simulink model "Glide_flare_alt"  (R2020a)
settings: Solver=VariableStepAuto  StartTime=0.0  StopTime=300  RelTol=1e-3
values from neighbouring files (symbols this model uses):
  A_reduced = A_lo([3,7,8,5,11],[3,7,8,5,11])    [landing.m]
  B_reduced = A_lo([3,7,8,5,11], [13,14])    [landing.m]
  C_reduced = C_lo([3,7,8,5,11],[3,7,8,5,11])    [landing.m]
  D_reduced = D_lo([3,7,8,5,11], [1,2])    [landing.m]
  elevator = -0.09    [FindF16Dynamics.m]    (also in runF16Sim.m; runLINF16sim.m)
  thrust = 5000    [FindF16Dynamics.m]    (also in landing.m = 2826.8165; runF16Sim.m; runLINF16sim.m = 0)
undefined symbols (not defined in the file or in its folder): magnitude
libraries: simulink_extras x5
settings Model: SnapshotBufferSize=10000  Creator=sarka  LastModifiedBy=mbrum

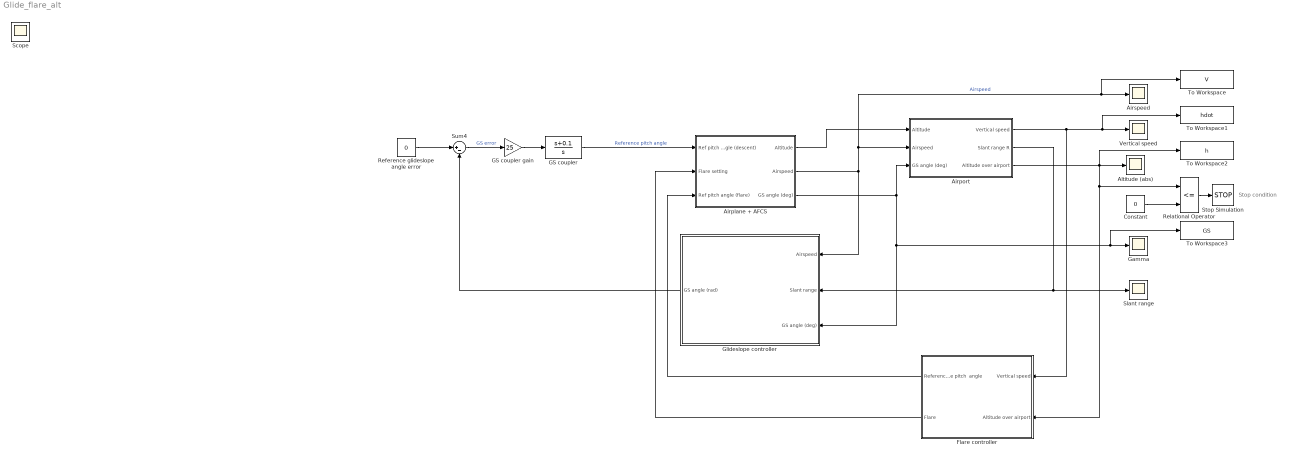
== system Glide_flare_alt ==
  note: Stop condition
  Airplane + AFCS : Subsystem
  Airport : Subsystem
  Airspeed : Scope
  Altitude (abs) : Scope
  Constant : Constant  Value=0
  Flare controller : Subsystem
  GS coupler : TransferFcn  Numerator=[1 0.1]  Denominator=[1 0]
  GS coupler gain : Gain  Gain=25
  Gamma : Scope
  Glideslope controller : Subsystem
  Reference glideslope angle error : Constant  Value=0
  Relational Operator : RelationalOperator  Operator=<=  OutDataTypeStr=boolean  RndMeth=Simplest
  Slant range : Scope
  Stop Simulation : Stop
  Sum4 : Sum  Inputs=|+-
  To Workspace : ToWorkspace  VariableName=V  SampleTime=-1
  To Workspace1 : ToWorkspace  VariableName=hdot  SampleTime=-1
  To Workspace2 : ToWorkspace  VariableName=h  SampleTime=-1
  To Workspace3 : ToWorkspace  VariableName=GS  SaveFormat=Timeseries  SampleTime=-1
  Vertical speed : Scope
  Scope : Scope
  wires:
  Airplane + AFCS/2(Airspeed) -> To Workspace/1, Airspeed/1, Airport/2(Airspeed), Glideslope controller/1(Airspeed)  "Airspeed"
  Airplane + AFCS/3(GS angle (deg)) -> Airport/3(GS angle (deg)), Glideslope controller/3(GS angle (deg)), To Workspace3/1, Gamma/1
  Airport/1(Vertical speed) -> To Workspace1/1, Vertical speed/1, Flare controller/1(Vertical speed)
  Reference glideslope angle error/1 -> Sum4/1
  Glideslope controller/1(GS angle (rad)) -> Sum4/2
  Sum4/1 -> GS coupler gain/1  "GS error"
  GS coupler gain/1 -> GS coupler/1
  Airplane + AFCS/1(Altitude) -> Airport/1(Altitude)
  Airport/2(Slant range R) -> Glideslope controller/2(Slant range), Slant range/1
  GS coupler/1 -> Airplane + AFCS/1(Ref pitch angle (descent))  "Reference pitch angle"
  Flare controller/2(Flare) -> Airplane + AFCS/2(Flare setting)
  Flare controller/1(Reference pitch  angle) -> Airplane + AFCS/3(Ref pitch angle (flare))
  Airport/3(Altitude over airport) -> To Workspace2/1, Flare controller/2(Altitude over airport), Relational Operator/1, Altitude (abs)/1
  Constant/1 -> Relational Operator/2
  Relational Operator/1 -> Stop Simulation/1

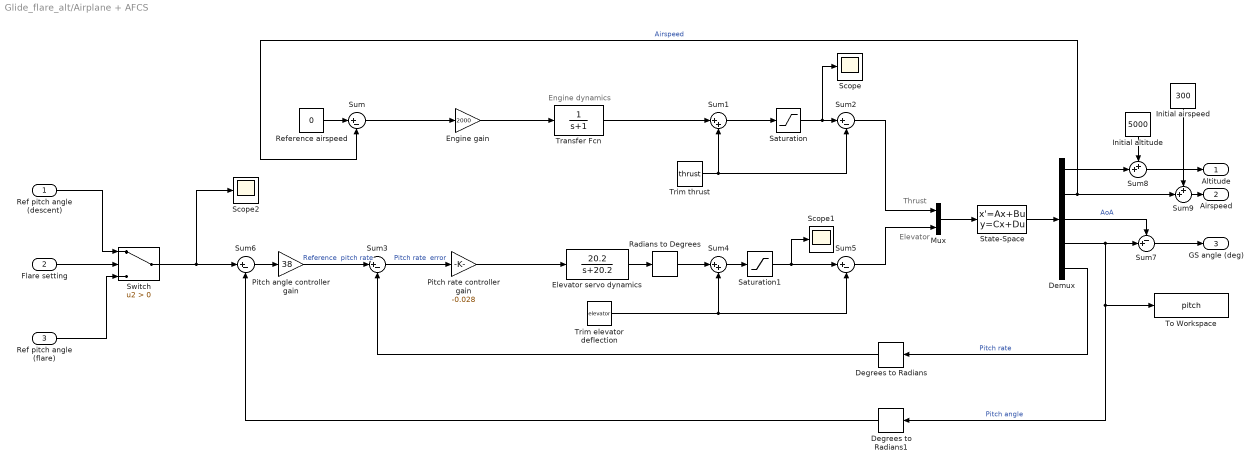
== system Glide_flare_alt/Airplane + AFCS ==
  note: Engine dynamics
  note: Elevator
  note: Thrust
  Ref pitch angle (descent) : Inport
  Flare setting : Inport  Port=2
  Ref pitch angle (flare) : Inport  Port=3
  Degrees to Radians : simulink_extras/Transformations/Degrees to Radians
  Degrees to Radians1 : simulink_extras/Transformations/Degrees to Radians
  Demux : Demux  Outputs=5
  Elevator servo dynamics : TransferFcn  Numerator=[20.2]  Denominator=[1 20.2]
  Engine gain : Gain  Gain=2000
  Initial airspeed : Constant  Value=300
  Initial altitude : Constant  Value=5000
  Mux : Mux  Inputs=2
  Pitch angle controller gain : Gain  Gain=38
  Pitch rate controller gain : Gain  Gain=-0.028
  Radians to Degrees : simulink_extras/Transformations/Radians to Degrees
  Reference airspeed : Constant  Value=0
  Saturation : Saturate  UpperLimit=19000  LowerLimit=1000
  Saturation1 : Saturate  UpperLimit=25  LowerLimit=-25
  Scope : Scope
  Scope1 : Scope
  Scope2 : Scope
  State-Space : StateSpace  A=A_reduced  B=B_reduced  C=C_reduced  D=D_reduced  InitialCondition=0
  Sum{,2..3,5..6} (5 alike) : Sum  Inputs=|+-
  Sum1 : Sum  Inputs=|++
  Sum4 : Sum  Inputs=|++
  Sum7 : Sum  Inputs=-+|
  Sum8 : Sum  Inputs=++|
  Sum9 : Sum  Inputs=++|
  Switch : Switch  Criteria=u2 > Threshold
  To Workspace : ToWorkspace  VariableName=pitch  SaveFormat=Timeseries  SampleTime=-1
  Transfer Fcn : TransferFcn  Denominator=[1 1]
  Trim elevator deflection : Constant  Value=elevator
  Trim thrust : Constant  Value=thrust
  Altitude : Outport
  Airspeed : Outport  Port=2
  GS angle (deg) : Outport  Port=3
  wires:
  Sum/1 -> Engine gain/1
  Radians to Degrees/1 -> Sum4/1
  Mux/1 -> State-Space/1
  Sum1/1 -> Saturation/1
  Pitch rate controller gain/1 -> Elevator servo dynamics/1
  Transfer Fcn/1 -> Sum1/1
  Sum4/1 -> Saturation1/1
  Elevator servo dynamics/1 -> Radians to Degrees/1
  Saturation/1 -> Scope/1, Sum2/1
  Sum2/1 -> Mux/1
  Trim elevator deflection/1 -> Sum4/2, Sum5/2
  Sum5/1 -> Mux/2
  Trim thrust/1 -> Sum2/2, Sum1/2
  Saturation1/1 -> Sum5/1, Scope1/1
  Reference airspeed/1 -> Sum/1
  Sum3/1 -> Pitch rate controller gain/1  "Pitch rate  error"
  Pitch angle controller gain/1 -> Sum3/1  "Reference  pitch rate"
  Engine gain/1 -> Transfer Fcn/1
  Demux/5 -> Degrees to Radians/1  "Pitch rate"
  Sum6/1 -> Pitch angle controller gain/1
  Demux/4 -> Degrees to Radians1/1, To Workspace/1, Sum7/2  "Pitch angle"
  State-Space/1 -> Demux/1
  Demux/3 -> Sum7/1  "AoA"
  Demux/1 -> Sum8/2
  Sum7/1 -> GS angle (deg)/1
  Degrees to Radians1/1 -> Sum6/2
  Degrees to Radians/1 -> Sum3/2
  Sum8/1 -> Altitude/1
  Initial altitude/1 -> Sum8/1
  Sum9/1 -> Airspeed/1
  Demux/2 -> Sum/2, Sum9/2  "Airspeed"
  Initial airspeed/1 -> Sum9/1
  Ref pitch angle (descent)/1 -> Switch/1
  Flare setting/1 -> Switch/2
  Ref pitch angle (flare)/1 -> Switch/3
  Switch/1 -> Scope2/1, Sum6/1

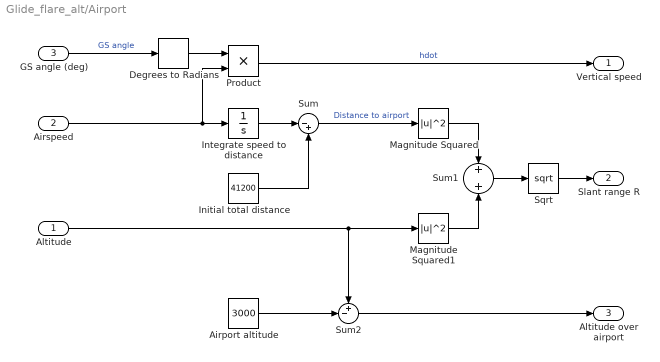
== system Glide_flare_alt/Airport ==
  Altitude : Inport
  Airspeed : Inport  Port=2
  GS angle (deg) : Inport  Port=3
  Airport altitude : Constant  Value=3000
  Degrees to Radians : simulink_extras/Transformations/Degrees to Radians
  Initial total distance : Constant  Value=41200
  Integrate speed to distance : Integrator
  Magnitude Squared : Math  Operator=magnitude^2  SaturateOnIntegerOverflow=on
  Magnitude Squared1 : Math  Operator=magnitude^2  SaturateOnIntegerOverflow=on
  Product : Product
  Sqrt : Sqrt  SaturateOnIntegerOverflow=on
  Sum : Sum  Inputs=|-+
  Sum1 : Sum  Inputs=+|+
  Sum2 : Sum  Inputs=+-|
  Vertical speed : Outport
  Slant range R : Outport  Port=2
  Altitude over airport : Outport  Port=3
  wires:
  GS angle (deg)/1 -> Degrees to Radians/1  "GS angle"
  Airspeed/1 -> Integrate speed to distance/1, Product/2
  Degrees to Radians/1 -> Product/1
  Product/1 -> Vertical speed/1  "hdot"
  Initial total distance/1 -> Sum/2
  Integrate speed to distance/1 -> Sum/1
  Sum/1 -> Magnitude Squared/1  "Distance to airport"
  Altitude/1 -> Sum2/1, Magnitude Squared1/1
  Sum1/1 -> Sqrt/1
  Magnitude Squared/1 -> Sum1/1
  Magnitude Squared1/1 -> Sum1/2
  Sqrt/1 -> Slant range R/1
  Airport altitude/1 -> Sum2/2
  Sum2/1 -> Altitude over airport/1

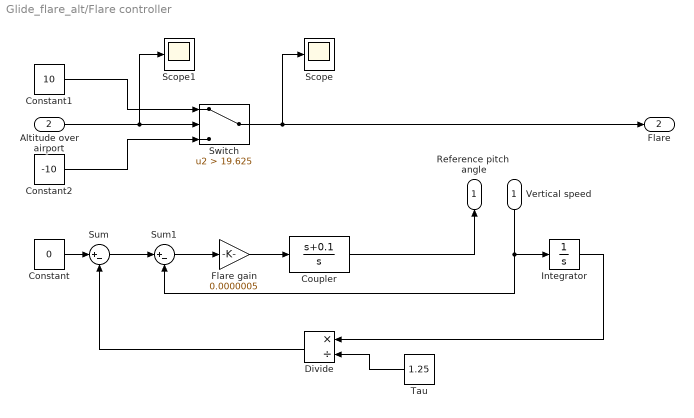
== system Glide_flare_alt/Flare controller ==
  Vertical speed : Inport
  Altitude over airport : Inport  Port=2
  Constant : Constant  Value=0
  Constant1 : Constant  Value=10
  Constant2 : Constant  Value=-10
  Coupler : TransferFcn  Numerator=[1 0.1]  Denominator=[1 0]
  Divide : Product  Inputs=*/
  Flare gain : Gain  Gain=0.0000005
  Integrator : Integrator
  Scope : Scope
  Scope1 : Scope
  Sum : Sum  Inputs=|+-
  Sum1 : Sum  Inputs=|+-
  Switch : Switch  Criteria=u2 > Threshold  Threshold=19.625
  Tau : Constant  Value=1.25
  Reference pitch  angle : Outport
  Flare : Outport  Port=2
  wires:
  Vertical speed/1 -> Sum1/2, Integrator/1
  Integrator/1 -> Divide/1
  Constant/1 -> Sum/1
  Sum/1 -> Sum1/1
  Flare gain/1 -> Coupler/1
  Sum1/1 -> Flare gain/1
  Coupler/1 -> Reference pitch  angle/1
  Altitude over airport/1 -> Scope1/1, Switch/2
  Constant1/1 -> Switch/1
  Constant2/1 -> Switch/3
  Switch/1 -> Scope/1, Flare/1
  Divide/1 -> Sum/2
  Tau/1 -> Divide/2

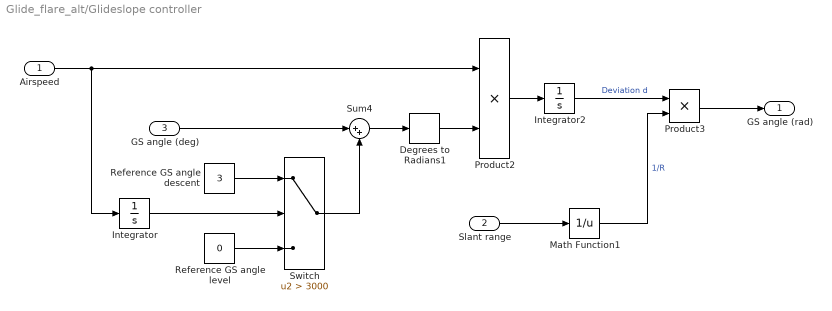
== system Glide_flare_alt/Glideslope controller ==
  Airspeed : Inport
  Slant range : Inport  Port=2
  GS angle (deg) : Inport  Port=3
  Degrees to Radians1 : simulink_extras/Transformations/Degrees to Radians
  Integrator : Integrator
  Integrator2 : Integrator
  Math Function1 : Math  Operator=reciprocal  SignedPower=on  RndMeth=Zero  SaturateOnIntegerOverflow=on
  Product2 : Product
  Product3 : Product
  Reference GS angle descent : Constant  Value=3
  Reference GS angle level : Constant  Value=0
  Sum4 : Sum  Inputs=|++
  Switch : Switch  Criteria=u2 > Threshold  Threshold=3000
  GS angle (rad) : Outport
  wires:
  GS angle (deg)/1 -> Sum4/1
  Reference GS angle level/1 -> Switch/3
  Sum4/1 -> Degrees to Radians1/1
  Airspeed/1 -> Integrator/1, Product2/1
  Product2/1 -> Integrator2/1
  Slant range/1 -> Math Function1/1
  Math Function1/1 -> Product3/2  "1/R"
  Integrator2/1 -> Product3/1  "Deviation d"
  Product3/1 -> GS angle (rad)/1
  Degrees to Radians1/1 -> Product2/2
  Reference GS angle descent/1 -> Switch/1
  Integrator/1 -> Switch/2
  Switch/1 -> Sum4/2
